simulink model "Attitude2sim"  (R2023b)
settings: Solver=VariableStepAuto  StartTime=0.0  StopTime=10.0  RelTol=1e-3
libraries: shared6dof x1
settings Model: Creator=jacksonwright  LastModifiedBy=jacksonwright

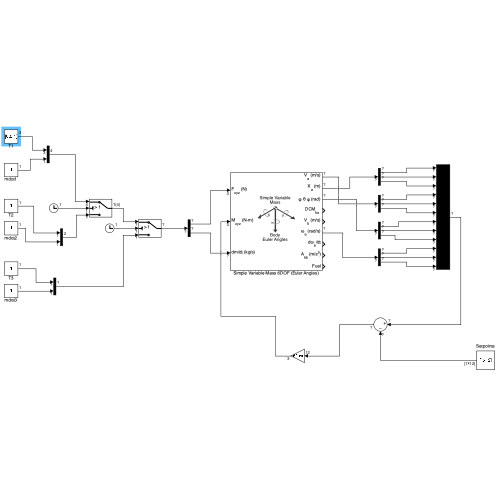
[thumbnail: Simulink's stored preview of the top-level diagram]
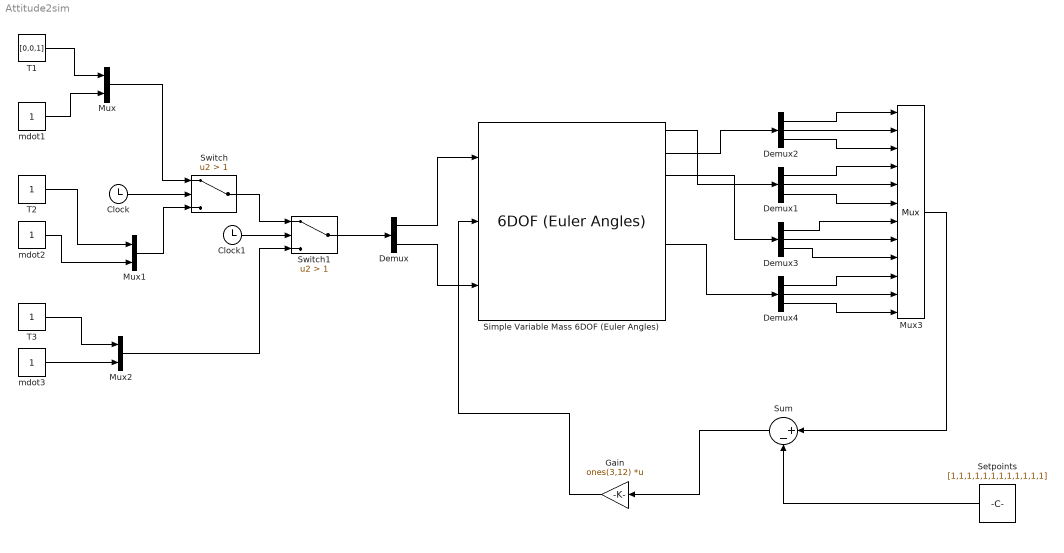
== system Attitude2sim ==
  Clock : Clock
  Clock1 : Clock
  Demux : Demux  Outputs=2
  Demux{1..4} (4 alike) : Demux  Outputs=3
  Gain : Gain  Gain=ones(3,12)  Multiplication=Matrix(K*u) (u vector)
  Mux : Mux  Inputs=2
  Mux1 : Mux  Inputs=2
  Mux2 : Mux  Inputs=2
  Mux3 : Mux  Inputs=12
  Setpoints : Constant  Value=[1,1,1,1,1,1,1,1,1,1,1,1]  VectorParams1D=off
  Simple Variable Mass 6DOF (Euler Angles) : shared6dof/6DOF (Euler Angles)  units=Metric (MKS)  mtype=Simple Variable  rep=Euler Angles  xme_0=[0 0 0]  Vm_0=[0 0 0]  eul_0=[0 0 0]  pm_0=[0 0 0]  mass_0=1.0  mass_e=0.5  mass_f=2.0  inertia=eye(3)  inertia_e=eye(3)  inertia_f=2*eye(3)  k_quat=1.0  vre_flag=off  abi_flag=off  aMode=0  xme_statename=''  Vm_statename=''  eul_statename=''  quat_statename=''  pm_statename=''  mass_statename=''
      settings: LibrarySourceBlock=aerolib6dof2/Simple Variable Mass 6DOF (Euler Angles)
  Sum : Sum  Inputs=|+-
  Switch : Switch  Criteria=u2 > Threshold  Threshold=1  SaturateOnIntegerOverflow=off  InputSameDT=off
  Switch1 : Switch  Criteria=u2 > Threshold  Threshold=1  SaturateOnIntegerOverflow=off  InputSameDT=off
  T1 : Constant  Value=[0,0,1]
  T2 : Constant
  T3 : Constant
  mdot1 : Constant
  mdot2 : Constant
  mdot3 : Constant
  wires:
  T1/1 -> Mux/1
  mdot1/1 -> Mux/2
  Mux/1 -> Switch/1
  Clock/1 -> Switch/2
  T2/1 -> Mux1/1
  mdot2/1 -> Mux1/2
  Mux1/1 -> Switch/3
  T3/1 -> Mux2/1
  mdot3/1 -> Mux2/2
  Mux2/1 -> Switch1/3
  Switch/1 -> Switch1/1
  Switch1/1 -> Demux/1
  Demux/1 -> Simple Variable Mass 6DOF (Euler Angles)/1
  Demux/2 -> Simple Variable Mass 6DOF (Euler Angles)/3
  Simple Variable Mass 6DOF (Euler Angles)/1 -> Demux1/1
  Demux1/1 -> Mux3/4
  Demux1/2 -> Mux3/5
  Demux1/3 -> Mux3/6
  Simple Variable Mass 6DOF (Euler Angles)/2 -> Demux2/1
  Demux2/2 -> Mux3/2
  Demux2/1 -> Mux3/1
  Demux2/3 -> Mux3/3
  Simple Variable Mass 6DOF (Euler Angles)/3 -> Demux3/1
  Demux3/1 -> Mux3/7
  Demux3/2 -> Mux3/8
  Demux3/3 -> Mux3/9
  Demux4/2 -> Mux3/11
  Demux4/1 -> Mux3/10
  Demux4/3 -> Mux3/12
  Simple Variable Mass 6DOF (Euler Angles)/6 -> Demux4/1
  Clock1/1 -> Switch1/2
  Mux3/1 -> Sum/1
  Setpoints/1 -> Sum/2
  Gain/1 -> Simple Variable Mass 6DOF (Euler Angles)/2
  Sum/1 -> Gain/1
